simulink model "aliasing_example"  (R2017a)
settings: Solver=ode45  StartTime=0.0  StopTime=40  RelTol=1e-3  EnableMultiTasking=on
values from neighbouring files (symbols this model uses):
  h = 2/10    (= 0.2)    [aliasing_example_model.m]    (also in notch_filter_example.m = 0.5; notch_filter_tustin_example.m = 0.5; sixty_hertz_hum_alias.m = 0.1)
  wralias = wN + (wN-wr)    (= 28.6659265359)    [aliasing_example_model.m]
undefined symbols (not defined in the file or in its folder): Fdden, Fdnum
settings Model: Creator=kjartan  LastModifiedBy=kjartan
settings DataIOCC: LimitDataPoints=on  SaveFormat=Array
settings OptimizationCC: LifeSpan=inf
settings DebuggingCC: SolverPrmCheckMsg=warning  SFUnexpectedBacktrackingDiag=warning  SFNoUnconditionalDefaultTransitionDiag=warning  SFExecutionAtInitializationDiag=none
settings HardwareCC: ProdBitPerPointer=32  ProdBitPerSizeT=32  ProdBitPerPtrDiffT=32  ProdLargestAtomicFloat=None  ProdIntDivRoundTo=Undefined  ProdEndianess=Unspecified  ProdWordSize=32  ProdHWDeviceType=32-bit Generic
settings ModelReferenceCC: PropagateSignalLabelsOutOfModel=off
settings GRTTargetCC: TargetLangStandard=C89/C90 (ANSI)  GeneratePreprocessorConditionals=Disable all
settings ConfigComp: CovMetricSettings=dw  CovHtmlReporting=on  CovSaveCumulativeToWorkspaceVar=on  CovSaveSingleToWorkspaceVar=on  CovExternalEMLEnable=off  CovSFcnEnable=off

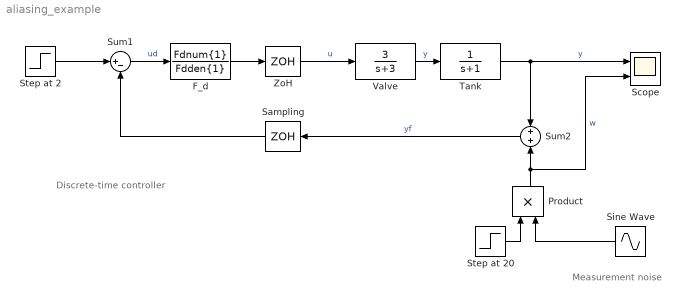
== system aliasing_example ==
  note: Measurement noise
  note: Discrete-time controller
  F_d : DiscreteTransferFcn  Numerator=Fdnum{1}  Denominator=Fdden{1}  SampleTime=h
  Product : Product
  Sampling : ZeroOrderHold  SampleTime=h
  Scope : Scope  NumInputPorts=2
  Sine Wave : Sin  Amplitude=0.05  Frequency=wralias  SampleTime=0
  Step at 2 : Step  Time=2  SampleTime=0
  Step at 20 : Step  Time=20  SampleTime=0
  Sum1 : Sum  Inputs=|+-
  Sum2 : Sum  Inputs=+|+
  Tank : TransferFcn  Denominator=[1 1]
  Valve : TransferFcn  Numerator=3  Denominator=[1, 3]
  ZoH : ZeroOrderHold  SampleTime=h
  wires:
  Sum1/1 -> F_d/1  "ud"
  Sampling/1 -> Sum1/2
  ZoH/1 -> Valve/1  "u"
  Step at 20/1 -> Product/1
  Product/1 -> Sum2/2, Scope/2  "w"
  Sum2/1 -> Sampling/1  "yf"
  Step at 2/1 -> Sum1/1
  F_d/1 -> ZoH/1
  Sine Wave/1 -> Product/2
  Valve/1 -> Tank/1  "y"
  Tank/1 -> Sum2/1, Scope/1  "y"
